simulink library "cylindricalPack_58kwhr_30Q_fade"  (R2025a)
settings: Solver=VariableStepAuto  StartTime=0.0  StopTime=10.0  RelTol=1e-3
undefined symbols (not defined in the file or in its folder): battery_builder_rtmsupport, gcbh
libraries: nesl_utility x75, cylindricalPack_58kwhr_30Q_fade_lib x36, batt_lib x1
(part 1 of 5)
settings Model: Creator=OADEBAJO  LastModifiedBy=OADEBAJO

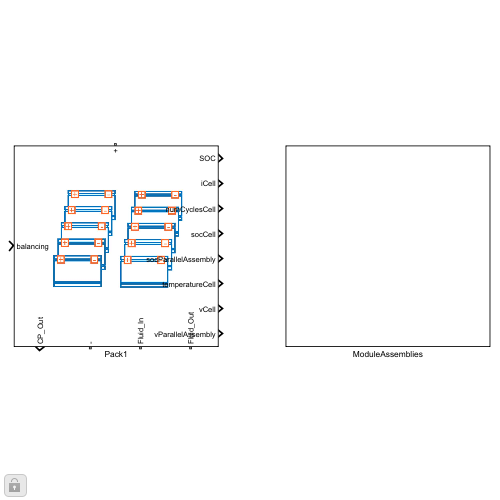
[thumbnail: Simulink's stored preview of the top-level diagram]
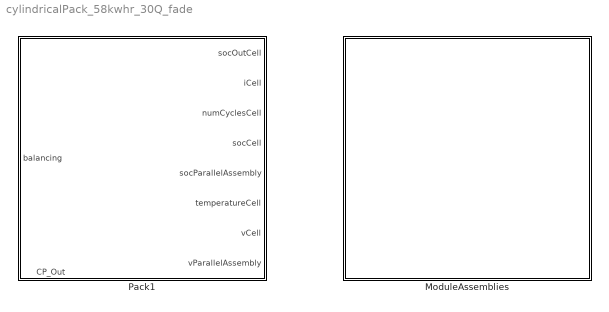
== system cylindricalPack_58kwhr_30Q_fade ==
  ModuleAssemblies : Subsystem
  Pack1 : Subsystem  LoadFcn=battery_builder_rtmsupport('loadfcn',gcbh);
      settings: CopyFcn=battery_builder_rtmsupport('copyfcn',gcbh);  PreCopyFcn=battery_builder_rtmsupport('precopyfcn',gcbh);  PreDeleteFcn=battery_builder_rtmsupport('predeletefcn',gcbh);  PortSchema="{\"entries\":[{\"content\":{\"sides\":[{\"content\":{\"connectorIds\":[\"LConn1\"]},\"type\":\"ConnectorPlacement.EquallySpacedRectSide\",\"uuid\":\"39220b85-9e56-421f-be99-25ff5c21c9d0\"},{\"content\":{\"connectorIds\":[\"Out1\",\"RConn1\",\"RConn2\",\"RConn3\"],\"side\":\"RIGHT\"},\"type\":\"ConnectorPlacement.EquallySpacedRectSide\",\"uuid\":\"8e68bd29-cf5f-450c-8507-e6fdf573813e\"},{\"content\":{\"connectorIds\":[\"In1\"],\"side\":\"TOP\"},\"type\":\"ConnectorPlacement.EquallySpacedRectSide\",\"uuid\":\"da231d6b-72d6-4d7b-b077-15d78428412a\"},{\"content\":{\"connectorIds\":[\"Out2\",\"Out3\",\"Out4\",\"Out5\",\"Out6\",\"Out7\",\"Out8\",\"Out9\"],\"side\":\"BOTTOM\"},\"type\":\"ConnectorPlacement.EquallySpacedRectSide\",\"uuid\":\"e98dc27c-cbdf-44be-82a1-87ffd4deded9\"}]},\"type\":\"ConnectorPlacement.EquallySpacedConnector\",\"uuid\":\"6b91b769-9080-486f-8a83-717e958640da\"}],\"packageUris\":[\"http://schema.mathworks.com/mf0/Connector/R2020b\"],\"version\":\"1.0\"}"
      mask Display: image('$imagefile')

== system cylindricalPack_58kwhr_30Q_fade/ModuleAssemblies ==
  ModuleAssemblyType1 : Subsystem  LoadFcn=battery_builder_rtmsupport('loadfcn',gcbh);
      settings: CopyFcn=battery_builder_rtmsupport('copyfcn',gcbh);  PreCopyFcn=battery_builder_rtmsupport('precopyfcn',gcbh);  PreDeleteFcn=battery_builder_rtmsupport('predeletefcn',gcbh);  PortSchema="{\"entries\":[{\"content\":{\"sides\":[{\"content\":{\"connectorIds\":[\"LConn1\"]},\"type\":\"ConnectorPlacement.EquallySpacedRectSide\",\"uuid\":\"edb2725c-ca29-40a6-9f70-0dabec9a46f5\"},{\"content\":{\"connectorIds\":[\"RConn1\",\"RConn2\"],\"side\":\"RIGHT\"},\"type\":\"ConnectorPlacement.EquallySpacedRectSide\",\"uuid\":\"4c0fe347-b718-4785-8871-63deed9ddb14\"},{\"content\":{\"connectorIds\":[\"In1\"],\"side\":\"TOP\"},\"type\":\"ConnectorPlacement.EquallySpacedRectSide\",\"uuid\":\"14c89690-db7b-421c-9ae6-2a7930fd5502\"},{\"content\":{\"connectorIds\":[\"Out1\",\"Out2\",\"Out3\",\"Out4\",\"Out5\",\"Out6\",\"Out7\",\"Out8\"],\"side\":\"BOTTOM\"},\"type\":\"ConnectorPlacement.EquallySpacedRectSide\",\"uuid\":\"cd90e9e9-4011-4b4d-baa7-3772b10580cf\"}]},\"type\":\"ConnectorPlacement.EquallySpacedConnector\",\"uuid\":\"bac0a601-b4a1-4bc6-ad24-9e7613281f89\"}],\"packageUris\":[\"http://schema.mathworks.com/mf0/Connector/R2020b\"],\"version\":\"1.0\"}"
      mask Display: image('$imagefile')
  ModuleAssemblyType2 : Subsystem  LoadFcn=battery_builder_rtmsupport('loadfcn',gcbh);
      settings: CopyFcn=battery_builder_rtmsupport('copyfcn',gcbh);  PreCopyFcn=battery_builder_rtmsupport('precopyfcn',gcbh);  PreDeleteFcn=battery_builder_rtmsupport('predeletefcn',gcbh);  PortSchema="{\"entries\":[{\"content\":{\"sides\":[{\"content\":{\"connectorIds\":[\"LConn1\"]},\"type\":\"ConnectorPlacement.EquallySpacedRectSide\",\"uuid\":\"edb2725c-ca29-40a6-9f70-0dabec9a46f5\"},{\"content\":{\"connectorIds\":[\"RConn1\",\"RConn2\"],\"side\":\"RIGHT\"},\"type\":\"ConnectorPlacement.EquallySpacedRectSide\",\"uuid\":\"4c0fe347-b718-4785-8871-63deed9ddb14\"},{\"content\":{\"connectorIds\":[\"In1\"],\"side\":\"TOP\"},\"type\":\"ConnectorPlacement.EquallySpacedRectSide\",\"uuid\":\"14c89690-db7b-421c-9ae6-2a7930fd5502\"},{\"content\":{\"connectorIds\":[\"Out1\",\"Out2\",\"Out3\",\"Out4\",\"Out5\",\"Out6\",\"Out7\",\"Out8\"],\"side\":\"BOTTOM\"},\"type\":\"ConnectorPlacement.EquallySpacedRectSide\",\"uuid\":\"26263ffa-138f-48ba-a92f-43b1044b6511\"}]},\"type\":\"ConnectorPlacement.EquallySpacedConnector\",\"uuid\":\"bac0a601-b4a1-4bc6-ad24-9e7613281f89\"}],\"packageUris\":[\"http://schema.mathworks.com/mf0/Connector/R2020b\"],\"version\":\"1.0\"}"
      mask Display: image('$imagefile')

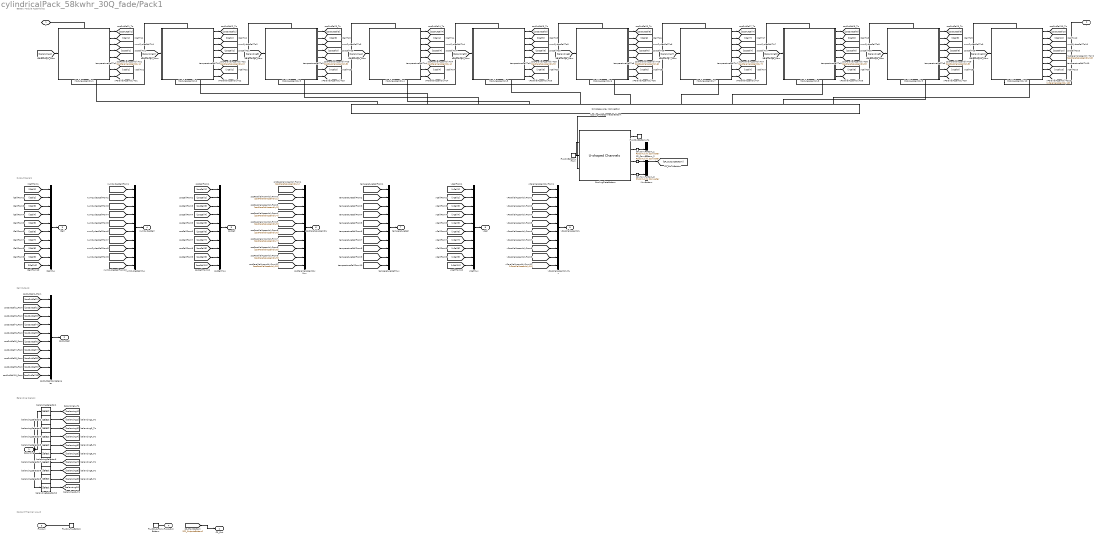
== system cylindricalPack_58kwhr_30Q_fade/Pack1 ==
  note: Battery Module Assemblies
  note: Output Signals
  note: Cell Outputs
  note: Balancing Signals
  note: Coolant Thermal Liquid
  balancing : Inport  PortDimensions=180
  CP_ConvBottom_1 : nesl_utility/PS-Simulink Converter  PhysicalDomain=network_engine_domain  SubClassName=ps_output  LeftPortType=input  RightPortType=output  PseudoPeriodic=off  Frequencies=[]  VectorFormat=inherit  Unit=inherit  AffineConversion=off
  CP_ConvBottom_2 : nesl_utility/PS-Simulink Converter  PhysicalDomain=network_engine_domain  SubClassName=ps_output  LeftPortType=input  RightPortType=output  PseudoPeriodic=off  Frequencies=[]  VectorFormat=inherit  Unit=inherit  AffineConversion=off
  CP_ConvBottom_3 : nesl_utility/PS-Simulink Converter  PhysicalDomain=network_engine_domain  SubClassName=ps_output  LeftPortType=input  RightPortType=output  PseudoPeriodic=off  Frequencies=[]  VectorFormat=inherit  Unit=inherit  AffineConversion=off
  CoolingPlateBottom : batt_lib/Thermal/U-shaped Channels  plateConnectivity=simscape.battery.enum.thermal.coolingPlateConnectivity.singleSided  numBattThermalNodes1=30  dimensionThermalNodes1=[[0.0955 0.7388;0.0955 0.7388;0.0955 0.7388;0.0955 0.7388;0.0955 0.7388;0.0955 0.7388;0.0955 0.7388;0.0955 0.7388;0.0955 0.7388;0.0955 0.7388;0.0955 0.7388;0.0955 0.7388;0.0955 0.7388;0.0955 0.7388;0.0955 0.7388;0.0955 0.7388;0.0955 0.7388;0.0955 0.7388;0.0955 0.7388;0.0955 0.7388;0.0955 0.7388;0.0955 0.7388;0.0955 0.7388;0.0955 0.7388;0.0955 0.7388;0.0955 0.7388;0.0955 0.7388;0.0955 0.7388;0.0955 0.7388;0.0955 0.7388]]  locationThermalNodes1=[[0.04775 0.3694;0.04775 0.3694;0.04775 0.3694;0.15325 0.3694;0.15325 0.3694;0.15325 0.3694;0.25875 0.3694;0.25875 0.3694;0.25875 0.3694;0.36425 0.3694;0.36425 0.3694;0.36425 0.3694;0.46975 0.3694;0.46975 0.3694;0.46975 0.3694;0.57525 0.3694;0.57525 0.3694;0.57525 0.3694;0.68075 0.3694;0.68075 0.3694;0.68075 0.3694;0.78625 0.3694;0.78625 0.3694;0.78625 0.3694;0.89175 0.3694;0.89175 0.3694;0.89175 0.3694;0.99725 0.3694;0.99725 0.3694;0.99725 0.3694]]  numBattThermalNodes2=1  dimensionThermalNodes2=ones(1, 2)  locationThermalNodes2=ones(1, 2)  plateDimX=2  plateDimY=5  plateTh=2e-3 m  plateThCond=20 W/(K*m)  plateDen=2500 kg/m^3  plateCp=447 J/(K*kg)  plateTemp_ini=300 K  Re_lam=2000  Re_tur=4000  Nu_lam=3.66  length_add=1e-3 m  shape_factor=64  nPartitions=1  selectChannelOrientation=simscape.battery.enum.thermal.coolingChannelsDirection.alongX  channelThickness=5e-03 m  barrierWidth=5e-03 m  roughnessPipe=1.5e-05 m
      settings: InternalSimscapePortConfiguration="{\"Bottom\":[],\"Left\":[{\"id\":\"fluid_in\",\"label\":\"fluid_in\",\"type\":\"foundation.thermal_liquid.thermal_liquid\"}],\"Right\":[{\"id\":\"fluid_out\",\"label\":\"fluid_out\",\"type\":\"foundation.thermal_liquid.thermal_liquid\"},{\"id\":\"plotPlateT\",\"label\":\"Tp\",\"type\":\"output\"},{\"id\":\"tempSensor\",\"label\":\"dT\",\"type\":\"output\"},{\"id\":\"presSensor\",\"label\":\"dP\",\"type\":\"output\"}],\"Top\":[{\"id\":\"Side1\",\"label\":\"Surf1\",\"type\":\"foundation.thermal.thermal\"}]}"
  CoolingPlateConnectorBottom : SimscapeArrayConnection  Domain=foundation.thermal.thermal  Mode=Sized Elements
  FluidInBottom_From : ConnectionLabel  Label=FluidIn_To_Bottom
  FluidIn_To_Bottom : ConnectionLabel  Label=FluidIn_To_Bottom
  FluidOutBottom_To : ConnectionLabel  Label=FluidOut_From_Bottom
  FluidOut_From_Bottom : ConnectionLabel  Label=FluidOut_From_Bottom
  ModuleAssembly1 : Subsystem  LoadFcn=battery_builder_rtmsupport('loadfcn',gcbh);
      settings: CopyFcn=battery_builder_rtmsupport('copyfcn',gcbh);  PreCopyFcn=battery_builder_rtmsupport('precopyfcn',gcbh);  PreDeleteFcn=battery_builder_rtmsupport('predeletefcn',gcbh);  PortSchema="{\"entries\":[{\"content\":{\"sides\":[{\"content\":{\"connectorIds\":[\"LConn1\"]},\"type\":\"ConnectorPlacement.EquallySpacedRectSide\",\"uuid\":\"edb2725c-ca29-40a6-9f70-0dabec9a46f5\"},{\"content\":{\"connectorIds\":[\"RConn1\",\"RConn2\"],\"side\":\"RIGHT\"},\"type\":\"ConnectorPlacement.EquallySpacedRectSide\",\"uuid\":\"4c0fe347-b718-4785-8871-63deed9ddb14\"},{\"content\":{\"connectorIds\":[\"In1\"],\"side\":\"TOP\"},\"type\":\"ConnectorPlacement.EquallySpacedRectSide\",\"uuid\":\"14c89690-db7b-421c-9ae6-2a7930fd5502\"},{\"content\":{\"connectorIds\":[\"Out1\",\"Out2\",\"Out3\",\"Out4\",\"Out5\",\"Out6\",\"Out7\",\"Out8\"],\"side\":\"BOTTOM\"},\"type\":\"ConnectorPlacement.EquallySpacedRectSide\",\"uuid\":\"cd90e9e9-4011-4b4d-baa7-3772b10580cf\"}]},\"type\":\"ConnectorPlacement.EquallySpacedConnector\",\"uuid\":\"bac0a601-b4a1-4bc6-ad24-9e7613281f89\"}],\"packageUris\":[\"http://schema.mathworks.com/mf0/Connector/R2020b\"],\"version\":\"1.0\"}"
      mask Display: image('$imagefile')
  ModuleAssembly10 : Subsystem  LoadFcn=battery_builder_rtmsupport('loadfcn',gcbh);
      settings: CopyFcn=battery_builder_rtmsupport('copyfcn',gcbh);  PreCopyFcn=battery_builder_rtmsupport('precopyfcn',gcbh);  PreDeleteFcn=battery_builder_rtmsupport('predeletefcn',gcbh);  PortSchema="{\"entries\":[{\"content\":{\"sides\":[{\"content\":{\"connectorIds\":[\"LConn1\"]},\"type\":\"ConnectorPlacement.EquallySpacedRectSide\",\"uuid\":\"edb2725c-ca29-40a6-9f70-0dabec9a46f5\"},{\"content\":{\"connectorIds\":[\"RConn1\",\"RConn2\"],\"side\":\"RIGHT\"},\"type\":\"ConnectorPlacement.EquallySpacedRectSide\",\"uuid\":\"4c0fe347-b718-4785-8871-63deed9ddb14\"},{\"content\":{\"connectorIds\":[\"In1\"],\"side\":\"TOP\"},\"type\":\"ConnectorPlacement.EquallySpacedRectSide\",\"uuid\":\"14c89690-db7b-421c-9ae6-2a7930fd5502\"},{\"content\":{\"connectorIds\":[\"Out1\",\"Out2\",\"Out3\",\"Out4\",\"Out5\",\"Out6\",\"Out7\",\"Out8\"],\"side\":\"BOTTOM\"},\"type\":\"ConnectorPlacement.EquallySpacedRectSide\",\"uuid\":\"26263ffa-138f-48ba-a92f-43b1044b6511\"}]},\"type\":\"ConnectorPlacement.EquallySpacedConnector\",\"uuid\":\"bac0a601-b4a1-4bc6-ad24-9e7613281f89\"}],\"packageUris\":[\"http://schema.mathworks.com/mf0/Connector/R2020b\"],\"version\":\"1.0\"}"
      mask Display: image('$imagefile')
  ModuleAssembly2 : Subsystem  LoadFcn=battery_builder_rtmsupport('loadfcn',gcbh);
      settings: CopyFcn=battery_builder_rtmsupport('copyfcn',gcbh);  PreCopyFcn=battery_builder_rtmsupport('precopyfcn',gcbh);  PreDeleteFcn=battery_builder_rtmsupport('predeletefcn',gcbh);  PortSchema="{\"entries\":[{\"content\":{\"sides\":[{\"content\":{\"connectorIds\":[\"LConn1\"]},\"type\":\"ConnectorPlacement.EquallySpacedRectSide\",\"uuid\":\"edb2725c-ca29-40a6-9f70-0dabec9a46f5\"},{\"content\":{\"connectorIds\":[\"RConn1\",\"RConn2\"],\"side\":\"RIGHT\"},\"type\":\"ConnectorPlacement.EquallySpacedRectSide\",\"uuid\":\"4c0fe347-b718-4785-8871-63deed9ddb14\"},{\"content\":{\"connectorIds\":[\"In1\"],\"side\":\"TOP\"},\"type\":\"ConnectorPlacement.EquallySpacedRectSide\",\"uuid\":\"14c89690-db7b-421c-9ae6-2a7930fd5502\"},{\"content\":{\"connectorIds\":[\"Out1\",\"Out2\",\"Out3\",\"Out4\",\"Out5\",\"Out6\",\"Out7\",\"Out8\"],\"side\":\"BOTTOM\"},\"type\":\"ConnectorPlacement.EquallySpacedRectSide\",\"uuid\":\"26263ffa-138f-48ba-a92f-43b1044b6511\"}]},\"type\":\"ConnectorPlacement.EquallySpacedConnector\",\"uuid\":\"bac0a601-b4a1-4bc6-ad24-9e7613281f89\"}],\"packageUris\":[\"http://schema.mathworks.com/mf0/Connector/R2020b\"],\"version\":\"1.0\"}"
      mask Display: image('$imagefile')
  ModuleAssembly3 : Subsystem  LoadFcn=battery_builder_rtmsupport('loadfcn',gcbh);
      settings: CopyFcn=battery_builder_rtmsupport('copyfcn',gcbh);  PreCopyFcn=battery_builder_rtmsupport('precopyfcn',gcbh);  PreDeleteFcn=battery_builder_rtmsupport('predeletefcn',gcbh);  PortSchema="{\"entries\":[{\"content\":{\"sides\":[{\"content\":{\"connectorIds\":[\"LConn1\"]},\"type\":\"ConnectorPlacement.EquallySpacedRectSide\",\"uuid\":\"edb2725c-ca29-40a6-9f70-0dabec9a46f5\"},{\"content\":{\"connectorIds\":[\"RConn1\",\"RConn2\"],\"side\":\"RIGHT\"},\"type\":\"ConnectorPlacement.EquallySpacedRectSide\",\"uuid\":\"4c0fe347-b718-4785-8871-63deed9ddb14\"},{\"content\":{\"connectorIds\":[\"In1\"],\"side\":\"TOP\"},\"type\":\"ConnectorPlacement.EquallySpacedRectSide\",\"uuid\":\"14c89690-db7b-421c-9ae6-2a7930fd5502\"},{\"content\":{\"connectorIds\":[\"Out1\",\"Out2\",\"Out3\",\"Out4\",\"Out5\",\"Out6\",\"Out7\",\"Out8\"],\"side\":\"BOTTOM\"},\"type\":\"ConnectorPlacement.EquallySpacedRectSide\",\"uuid\":\"26263ffa-138f-48ba-a92f-43b1044b6511\"}]},\"type\":\"ConnectorPlacement.EquallySpacedConnector\",\"uuid\":\"bac0a601-b4a1-4bc6-ad24-9e7613281f89\"}],\"packageUris\":[\"http://schema.mathworks.com/mf0/Connector/R2020b\"],\"version\":\"1.0\"}"
      mask Display: image('$imagefile')
  ModuleAssembly4 : Subsystem  LoadFcn=battery_builder_rtmsupport('loadfcn',gcbh);
      settings: CopyFcn=battery_builder_rtmsupport('copyfcn',gcbh);  PreCopyFcn=battery_builder_rtmsupport('precopyfcn',gcbh);  PreDeleteFcn=battery_builder_rtmsupport('predeletefcn',gcbh);  PortSchema="{\"entries\":[{\"content\":{\"sides\":[{\"content\":{\"connectorIds\":[\"LConn1\"]},\"type\":\"ConnectorPlacement.EquallySpacedRectSide\",\"uuid\":\"edb2725c-ca29-40a6-9f70-0dabec9a46f5\"},{\"content\":{\"connectorIds\":[\"RConn1\",\"RConn2\"],\"side\":\"RIGHT\"},\"type\":\"ConnectorPlacement.EquallySpacedRectSide\",\"uuid\":\"4c0fe347-b718-4785-8871-63deed9ddb14\"},{\"content\":{\"connectorIds\":[\"In1\"],\"side\":\"TOP\"},\"type\":\"ConnectorPlacement.EquallySpacedRectSide\",\"uuid\":\"14c89690-db7b-421c-9ae6-2a7930fd5502\"},{\"content\":{\"connectorIds\":[\"Out1\",\"Out2\",\"Out3\",\"Out4\",\"Out5\",\"Out6\",\"Out7\",\"Out8\"],\"side\":\"BOTTOM\"},\"type\":\"ConnectorPlacement.EquallySpacedRectSide\",\"uuid\":\"26263ffa-138f-48ba-a92f-43b1044b6511\"}]},\"type\":\"ConnectorPlacement.EquallySpacedConnector\",\"uuid\":\"bac0a601-b4a1-4bc6-ad24-9e7613281f89\"}],\"packageUris\":[\"http://schema.mathworks.com/mf0/Connector/R2020b\"],\"version\":\"1.0\"}"
      mask Display: image('$imagefile')
  ModuleAssembly5 : Subsystem  LoadFcn=battery_builder_rtmsupport('loadfcn',gcbh);
      settings: CopyFcn=battery_builder_rtmsupport('copyfcn',gcbh);  PreCopyFcn=battery_builder_rtmsupport('precopyfcn',gcbh);  PreDeleteFcn=battery_builder_rtmsupport('predeletefcn',gcbh);  PortSchema="{\"entries\":[{\"content\":{\"sides\":[{\"content\":{\"connectorIds\":[\"LConn1\"]},\"type\":\"ConnectorPlacement.EquallySpacedRectSide\",\"uuid\":\"edb2725c-ca29-40a6-9f70-0dabec9a46f5\"},{\"content\":{\"connectorIds\":[\"RConn1\",\"RConn2\"],\"side\":\"RIGHT\"},\"type\":\"ConnectorPlacement.EquallySpacedRectSide\",\"uuid\":\"4c0fe347-b718-4785-8871-63deed9ddb14\"},{\"content\":{\"connectorIds\":[\"In1\"],\"side\":\"TOP\"},\"type\":\"ConnectorPlacement.EquallySpacedRectSide\",\"uuid\":\"14c89690-db7b-421c-9ae6-2a7930fd5502\"},{\"content\":{\"connectorIds\":[\"Out1\",\"Out2\",\"Out3\",\"Out4\",\"Out5\",\"Out6\",\"Out7\",\"Out8\"],\"side\":\"BOTTOM\"},\"type\":\"ConnectorPlacement.EquallySpacedRectSide\",\"uuid\":\"26263ffa-138f-48ba-a92f-43b1044b6511\"}]},\"type\":\"ConnectorPlacement.EquallySpacedConnector\",\"uuid\":\"bac0a601-b4a1-4bc6-ad24-9e7613281f89\"}],\"packageUris\":[\"http://schema.mathworks.com/mf0/Connector/R2020b\"],\"version\":\"1.0\"}"
      mask Display: image('$imagefile')
  ModuleAssembly6 : Subsystem  LoadFcn=battery_builder_rtmsupport('loadfcn',gcbh);
      settings: CopyFcn=battery_builder_rtmsupport('copyfcn',gcbh);  PreCopyFcn=battery_builder_rtmsupport('precopyfcn',gcbh);  PreDeleteFcn=battery_builder_rtmsupport('predeletefcn',gcbh);  PortSchema="{\"entries\":[{\"content\":{\"sides\":[{\"content\":{\"connectorIds\":[\"LConn1\"]},\"type\":\"ConnectorPlacement.EquallySpacedRectSide\",\"uuid\":\"edb2725c-ca29-40a6-9f70-0dabec9a46f5\"},{\"content\":{\"connectorIds\":[\"RConn1\",\"RConn2\"],\"side\":\"RIGHT\"},\"type\":\"ConnectorPlacement.EquallySpacedRectSide\",\"uuid\":\"4c0fe347-b718-4785-8871-63deed9ddb14\"},{\"content\":{\"connectorIds\":[\"In1\"],\"side\":\"TOP\"},\"type\":\"ConnectorPlacement.EquallySpacedRectSide\",\"uuid\":\"14c89690-db7b-421c-9ae6-2a7930fd5502\"},{\"content\":{\"connectorIds\":[\"Out1\",\"Out2\",\"Out3\",\"Out4\",\"Out5\",\"Out6\",\"Out7\",\"Out8\"],\"side\":\"BOTTOM\"},\"type\":\"ConnectorPlacement.EquallySpacedRectSide\",\"uuid\":\"26263ffa-138f-48ba-a92f-43b1044b6511\"}]},\"type\":\"ConnectorPlacement.EquallySpacedConnector\",\"uuid\":\"bac0a601-b4a1-4bc6-ad24-9e7613281f89\"}],\"packageUris\":[\"http://schema.mathworks.com/mf0/Connector/R2020b\"],\"version\":\"1.0\"}"
      mask Display: image('$imagefile')
  ModuleAssembly7 : Subsystem  LoadFcn=battery_builder_rtmsupport('loadfcn',gcbh);
      settings: CopyFcn=battery_builder_rtmsupport('copyfcn',gcbh);  PreCopyFcn=battery_builder_rtmsupport('precopyfcn',gcbh);  PreDeleteFcn=battery_builder_rtmsupport('predeletefcn',gcbh);  PortSchema="{\"entries\":[{\"content\":{\"sides\":[{\"content\":{\"connectorIds\":[\"LConn1\"]},\"type\":\"ConnectorPlacement.EquallySpacedRectSide\",\"uuid\":\"edb2725c-ca29-40a6-9f70-0dabec9a46f5\"},{\"content\":{\"connectorIds\":[\"RConn1\",\"RConn2\"],\"side\":\"RIGHT\"},\"type\":\"ConnectorPlacement.EquallySpacedRectSide\",\"uuid\":\"4c0fe347-b718-4785-8871-63deed9ddb14\"},{\"content\":{\"connectorIds\":[\"In1\"],\"side\":\"TOP\"},\"type\":\"ConnectorPlacement.EquallySpacedRectSide\",\"uuid\":\"14c89690-db7b-421c-9ae6-2a7930fd5502\"},{\"content\":{\"connectorIds\":[\"Out1\",\"Out2\",\"Out3\",\"Out4\",\"Out5\",\"Out6\",\"Out7\",\"Out8\"],\"side\":\"BOTTOM\"},\"type\":\"ConnectorPlacement.EquallySpacedRectSide\",\"uuid\":\"26263ffa-138f-48ba-a92f-43b1044b6511\"}]},\"type\":\"ConnectorPlacement.EquallySpacedConnector\",\"uuid\":\"bac0a601-b4a1-4bc6-ad24-9e7613281f89\"}],\"packageUris\":[\"http://schema.mathworks.com/mf0/Connector/R2020b\"],\"version\":\"1.0\"}"
      mask Display: image('$imagefile')
  ModuleAssembly8 : Subsystem  LoadFcn=battery_builder_rtmsupport('loadfcn',gcbh);
      settings: CopyFcn=battery_builder_rtmsupport('copyfcn',gcbh);  PreCopyFcn=battery_builder_rtmsupport('precopyfcn',gcbh);  PreDeleteFcn=battery_builder_rtmsupport('predeletefcn',gcbh);  PortSchema="{\"entries\":[{\"content\":{\"sides\":[{\"content\":{\"connectorIds\":[\"LConn1\"]},\"type\":\"ConnectorPlacement.EquallySpacedRectSide\",\"uuid\":\"edb2725c-ca29-40a6-9f70-0dabec9a46f5\"},{\"content\":{\"connectorIds\":[\"RConn1\",\"RConn2\"],\"side\":\"RIGHT\"},\"type\":\"ConnectorPlacement.EquallySpacedRectSide\",\"uuid\":\"4c0fe347-b718-4785-8871-63deed9ddb14\"},{\"content\":{\"connectorIds\":[\"In1\"],\"side\":\"TOP\"},\"type\":\"ConnectorPlacement.EquallySpacedRectSide\",\"uuid\":\"14c89690-db7b-421c-9ae6-2a7930fd5502\"},{\"content\":{\"connectorIds\":[\"Out1\",\"Out2\",\"Out3\",\"Out4\",\"Out5\",\"Out6\",\"Out7\",\"Out8\"],\"side\":\"BOTTOM\"},\"type\":\"ConnectorPlacement.EquallySpacedRectSide\",\"uuid\":\"26263ffa-138f-48ba-a92f-43b1044b6511\"}]},\"type\":\"ConnectorPlacement.EquallySpacedConnector\",\"uuid\":\"bac0a601-b4a1-4bc6-ad24-9e7613281f89\"}],\"packageUris\":[\"http://schema.mathworks.com/mf0/Connector/R2020b\"],\"version\":\"1.0\"}"
      mask Display: image('$imagefile')
  ModuleAssembly9 : Subsystem  LoadFcn=battery_builder_rtmsupport('loadfcn',gcbh);
      settings: CopyFcn=battery_builder_rtmsupport('copyfcn',gcbh);  PreCopyFcn=battery_builder_rtmsupport('precopyfcn',gcbh);  PreDeleteFcn=battery_builder_rtmsupport('predeletefcn',gcbh);  PortSchema="{\"entries\":[{\"content\":{\"sides\":[{\"content\":{\"connectorIds\":[\"LConn1\"]},\"type\":\"ConnectorPlacement.EquallySpacedRectSide\",\"uuid\":\"edb2725c-ca29-40a6-9f70-0dabec9a46f5\"},{\"content\":{\"connectorIds\":[\"RConn1\",\"RConn2\"],\"side\":\"RIGHT\"},\"type\":\"ConnectorPlacement.EquallySpacedRectSide\",\"uuid\":\"4c0fe347-b718-4785-8871-63deed9ddb14\"},{\"content\":{\"connectorIds\":[\"In1\"],\"side\":\"TOP\"},\"type\":\"ConnectorPlacement.EquallySpacedRectSide\",\"uuid\":\"14c89690-db7b-421c-9ae6-2a7930fd5502\"},{\"content\":{\"connectorIds\":[\"Out1\",\"Out2\",\"Out3\",\"Out4\",\"Out5\",\"Out6\",\"Out7\",\"Out8\"],\"side\":\"BOTTOM\"},\"type\":\"ConnectorPlacement.EquallySpacedRectSide\",\"uuid\":\"26263ffa-138f-48ba-a92f-43b1044b6511\"}]},\"type\":\"ConnectorPlacement.EquallySpacedConnector\",\"uuid\":\"bac0a601-b4a1-4bc6-ad24-9e7613281f89\"}],\"packageUris\":[\"http://schema.mathworks.com/mf0/Connector/R2020b\"],\"version\":\"1.0\"}"
      mask Display: image('$imagefile')
  MuxBottom : Mux  Inputs=3
  balancingSelector1 : Selector  InputPortWidth=180  IndexOptions=Index vector (dialog)  Indices="[1   2   3   4   5   6   7   8   9  10  11  12  13  14  15  16  17  18]"  OutputSizes=1
  balancingSelector10 : Selector  InputPortWidth=180  IndexOptions=Index vector (dialog)  Indices="[163  164  165  166  167  168  169  170  171  172  173  174  175  176  177  178  179  180]"  OutputSizes=1
  balancingSelector2 : Selector  InputPortWidth=180  IndexOptions=Index vector (dialog)  Indices="[19  20  21  22  23  24  25  26  27  28  29  30  31  32  33  34  35  36]"  OutputSizes=1
  balancingSelector3 : Selector  InputPortWidth=180  IndexOptions=Index vector (dialog)  Indices="[37  38  39  40  41  42  43  44  45  46  47  48  49  50  51  52  53  54]"  OutputSizes=1
  balancingSelector4 : Selector  InputPortWidth=180  IndexOptions=Index vector (dialog)  Indices="[55  56  57  58  59  60  61  62  63  64  65  66  67  68  69  70  71  72]"  OutputSizes=1
  balancingSelector5 : Selector  InputPortWidth=180  IndexOptions=Index vector (dialog)  Indices="[73  74  75  76  77  78  79  80  81  82  83  84  85  86  87  88  89  90]"  OutputSizes=1
  balancingSelector6 : Selector  InputPortWidth=180  IndexOptions=Index vector (dialog)  Indices="[91   92   93   94   95   96   97   98   99  100  101  102  103  104  105  106  107  108]"  OutputSizes=1
  balancingSelector7 : Selector  InputPortWidth=180  IndexOptions=Index vector (dialog)  Indices="[109  110  111  112  113  114  115  116  117  118  119  120  121  122  123  124  125  126]"  OutputSizes=1
  balancingSelector8 : Selector  InputPortWidth=180  IndexOptions=Index vector (dialog)  Indices="[127  128  129  130  131  132  133  134  135  136  137  138  139  140  141  142  143  144]"  OutputSizes=1
  balancingSelector9 : Selector  InputPortWidth=180  IndexOptions=Index vector (dialog)  Indices="[145  146  147  148  149  150  151  152  153  154  155  156  157  158  159  160  161  162]"  OutputSizes=1
  iCellMux : Mux  Inputs=10
  numCyclesCellMux : Mux  Inputs=10
  socCellMux : Mux  Inputs=10
  socOutCellConcatenate : Concatenate  NumInputs=10  Mode=Multidimensional array  ConcatenateDimension=2
  socParallelAssemblyMux : Mux  Inputs=10
  temperatureCellMux : Mux  Inputs=10
  vCellMux : Mux  Inputs=10
  vParallelAssemblyMux : Mux  Inputs=10
  + : PMIOPort  Side=Left
  - : PMIOPort  Port=2  Side=Right
  Fluid_In : PMIOPort  Port=3  Side=Right  ConnectionType=Connection: foundation.thermal_liquid.thermal_liquid
  Fluid_Out : PMIOPort  Port=4  Side=Right  ConnectionType=Connection: foundation.thermal_liquid.thermal_liquid
  CP_Out : Outport
  socOutCell : Outport  Port=2
  iCell : Outport  Port=3
  numCyclesCell : Outport  Port=4
  socCell : Outport  Port=5
  socParallelAssembly : Outport  Port=6
  temperatureCell : Outport  Port=7
  vCell : Outport  Port=8
  vParallelAssembly : Outport  Port=9
  wires:
  socOutCellConcatenate/1 -> socOutCell/1  "SOC"
  [socOutCell1] -> socOutCellConcatenate/1
  [socOutCell2] -> socOutCellConcatenate/2
  [socOutCell3] -> socOutCellConcatenate/3
  [socOutCell4] -> socOutCellConcatenate/4
  [socOutCell5] -> socOutCellConcatenate/5
  [socOutCell6] -> socOutCellConcatenate/6
  [socOutCell7] -> socOutCellConcatenate/7
  [socOutCell8] -> socOutCellConcatenate/8
  [socOutCell9] -> socOutCellConcatenate/9
  [socOutCell10] -> socOutCellConcatenate/10
  ModuleAssembly1/2(iCell) -> [iCell1]
  iCellMux/1 -> iCell/1
  [iCell1] -> iCellMux/1
  ModuleAssembly1/3(numCyclesCell) -> [numCyclesCell1]
  numCyclesCellMux/1 -> numCyclesCell/1
  [numCyclesCell1] -> numCyclesCellMux/1
  ModuleAssembly1/4(socCell) -> [socCell1]
  socCellMux/1 -> socCell/1
  [socCell1] -> socCellMux/1
  ModuleAssembly1/5(socParallelAssembly) -> [socParallelAssembly1]
  socParallelAssemblyMux/1 -> socParallelAssembly/1
  [socParallelAssembly1] -> socParallelAssemblyMux/1
  ModuleAssembly1/6(temperatureCell) -> [temperatureCell1]
  temperatureCellMux/1 -> temperatureCell/1
  [temperatureCell1] -> temperatureCellMux/1
  ModuleAssembly1/7(vCell) -> [vCell1]
  vCellMux/1 -> vCell/1
  [vCell1] -> vCellMux/1
  ModuleAssembly1/8(vParallelAssembly) -> [vParallelAssembly1]
  vParallelAssemblyMux/1 -> vParallelAssembly/1
  [vParallelAssembly1] -> vParallelAssemblyMux/1
  ModuleAssembly2/2(iCell) -> [iCell2]
  [iCell2] -> iCellMux/2
  ModuleAssembly2/3(numCyclesCell) -> [numCyclesCell2]
  [numCyclesCell2] -> numCyclesCellMux/2
  ModuleAssembly2/4(socCell) -> [socCell2]
  [socCell2] -> socCellMux/2
  ModuleAssembly2/5(socParallelAssembly) -> [socParallelAssembly2]
  [socParallelAssembly2] -> socParallelAssemblyMux/2
  ModuleAssembly2/6(temperatureCell) -> [temperatureCell2]
  [temperatureCell2] -> temperatureCellMux/2
  ModuleAssembly2/7(vCell) -> [vCell2]
  [vCell2] -> vCellMux/2
  ModuleAssembly2/8(vParallelAssembly) -> [vParallelAssembly2]
  [vParallelAssembly2] -> vParallelAssemblyMux/2
  ModuleAssembly3/2(iCell) -> [iCell3]
  [iCell3] -> iCellMux/3
  ModuleAssembly3/3(numCyclesCell) -> [numCyclesCell3]
  [numCyclesCell3] -> numCyclesCellMux/3
  ModuleAssembly3/4(socCell) -> [socCell3]
  [socCell3] -> socCellMux/3
  ModuleAssembly3/5(socParallelAssembly) -> [socParallelAssembly3]
  [socParallelAssembly3] -> socParallelAssemblyMux/3
  ModuleAssembly3/6(temperatureCell) -> [temperatureCell3]
  [temperatureCell3] -> temperatureCellMux/3
  ModuleAssembly3/7(vCell) -> [vCell3]
  [vCell3] -> vCellMux/3
  ModuleAssembly3/8(vParallelAssembly) -> [vParallelAssembly3]
  [vParallelAssembly3] -> vParallelAssemblyMux/3
  ModuleAssembly4/2(iCell) -> [iCell4]
  [iCell4] -> iCellMux/4
  ModuleAssembly4/3(numCyclesCell) -> [numCyclesCell4]
  [numCyclesCell4] -> numCyclesCellMux/4
  ModuleAssembly4/4(socCell) -> [socCell4]
  [socCell4] -> socCellMux/4
  ModuleAssembly4/5(socParallelAssembly) -> [socParallelAssembly4]
  [socParallelAssembly4] -> socParallelAssemblyMux/4
  ModuleAssembly4/6(temperatureCell) -> [temperatureCell4]
  [temperatureCell4] -> temperatureCellMux/4
  ModuleAssembly4/7(vCell) -> [vCell4]
  [vCell4] -> vCellMux/4
  ModuleAssembly4/8(vParallelAssembly) -> [vParallelAssembly4]
  [vParallelAssembly4] -> vParallelAssemblyMux/4
  ModuleAssembly5/2(iCell) -> [iCell5]
  [iCell5] -> iCellMux/5
  ModuleAssembly5/3(numCyclesCell) -> [numCyclesCell5]
  [numCyclesCell5] -> numCyclesCellMux/5
  ModuleAssembly5/4(socCell) -> [socCell5]
  [socCell5] -> socCellMux/5
  ModuleAssembly5/5(socParallelAssembly) -> [socParallelAssembly5]
  [socParallelAssembly5] -> socParallelAssemblyMux/5
  ModuleAssembly5/6(temperatureCell) -> [temperatureCell5]
  [temperatureCell5] -> temperatureCellMux/5
  ModuleAssembly5/7(vCell) -> [vCell5]
  [vCell5] -> vCellMux/5
  ModuleAssembly5/8(vParallelAssembly) -> [vParallelAssembly5]
  [vParallelAssembly5] -> vParallelAssemblyMux/5
  ModuleAssembly6/2(iCell) -> [iCell6]
  [iCell6] -> iCellMux/6
  ModuleAssembly6/3(numCyclesCell) -> [numCyclesCell6]
  [numCyclesCell6] -> numCyclesCellMux/6
  ModuleAssembly6/4(socCell) -> [socCell6]
  [socCell6] -> socCellMux/6
  ModuleAssembly6/5(socParallelAssembly) -> [socParallelAssembly6]
  [socParallelAssembly6] -> socParallelAssemblyMux/6
  ModuleAssembly6/6(temperatureCell) -> [temperatureCell6]
  [temperatureCell6] -> temperatureCellMux/6
  ModuleAssembly6/7(vCell) -> [vCell6]
  [vCell6] -> vCellMux/6
  ModuleAssembly6/8(vParallelAssembly) -> [vParallelAssembly6]
  [vParallelAssembly6] -> vParallelAssemblyMux/6
  ModuleAssembly7/2(iCell) -> [iCell7]
  [iCell7] -> iCellMux/7
  ModuleAssembly7/3(numCyclesCell) -> [numCyclesCell7]
  [numCyclesCell7] -> numCyclesCellMux/7
  ModuleAssembly7/4(socCell) -> [socCell7]
  [socCell7] -> socCellMux/7
  ModuleAssembly7/5(socParallelAssembly) -> [socParallelAssembly7]
  [socParallelAssembly7] -> socParallelAssemblyMux/7
  ModuleAssembly7/6(temperatureCell) -> [temperatureCell7]
  [temperatureCell7] -> temperatureCellMux/7
  ModuleAssembly7/7(vCell) -> [vCell7]
  [vCell7] -> vCellMux/7
  ModuleAssembly7/8(vParallelAssembly) -> [vParallelAssembly7]
  [vParallelAssembly7] -> vParallelAssemblyMux/7
  ModuleAssembly8/2(iCell) -> [iCell8]
  [iCell8] -> iCellMux/8
  ModuleAssembly8/3(numCyclesCell) -> [numCyclesCell8]
  [numCyclesCell8] -> numCyclesCellMux/8
  ModuleAssembly8/4(socCell) -> [socCell8]
  [socCell8] -> socCellMux/8
  ModuleAssembly8/5(socParallelAssembly) -> [socParallelAssembly8]
  [socParallelAssembly8] -> socParallelAssemblyMux/8
  ModuleAssembly8/6(temperatureCell) -> [temperatureCell8]
  [temperatureCell8] -> temperatureCellMux/8
  ModuleAssembly8/7(vCell) -> [vCell8]
  [vCell8] -> vCellMux/8
  ModuleAssembly8/8(vParallelAssembly) -> [vParallelAssembly8]
  [vParallelAssembly8] -> vParallelAssemblyMux/8
  ModuleAssembly9/2(iCell) -> [iCell9]
  [iCell9] -> iCellMux/9
  ModuleAssembly9/3(numCyclesCell) -> [numCyclesCell9]
  [numCyclesCell9] -> numCyclesCellMux/9
  ModuleAssembly9/4(socCell) -> [socCell9]
  [socCell9] -> socCellMux/9
  ModuleAssembly9/5(socParallelAssembly) -> [socParallelAssembly9]
  [socParallelAssembly9] -> socParallelAssemblyMux/9
  ModuleAssembly9/6(temperatureCell) -> [temperatureCell9]
  [temperatureCell9] -> temperatureCellMux/9
  ModuleAssembly9/7(vCell) -> [vCell9]
  [vCell9] -> vCellMux/9
  ModuleAssembly9/8(vParallelAssembly) -> [vParallelAssembly9]
  [vParallelAssembly9] -> vParallelAssemblyMux/9
  ModuleAssembly10/2(iCell) -> [iCell10]
  [iCell10] -> iCellMux/10
  ModuleAssembly10/3(numCyclesCell) -> [numCyclesCell10]
  [numCyclesCell10] -> numCyclesCellMux/10
  ModuleAssembly10/4(socCell) -> [socCell10]
  [socCell10] -> socCellMux/10
  ModuleAssembly10/5(socParallelAssembly) -> [socParallelAssembly10]
  [socParallelAssembly10] -> socParallelAssemblyMux/10
  ModuleAssembly10/6(temperatureCell) -> [temperatureCell10]
  [temperatureCell10] -> temperatureCellMux/10
  ModuleAssembly10/7(vCell) -> [vCell10]
  [vCell10] -> vCellMux/10
  ModuleAssembly10/8(vParallelAssembly) -> [vParallelAssembly10]
  [vParallelAssembly10] -> vParallelAssemblyMux/10
  ModuleAssembly1/1(socOutCell) -> [socOutCell1]
  ModuleAssembly2/1(socOutCell) -> [socOutCell2]
  ModuleAssembly3/1(socOutCell) -> [socOutCell3]
  ModuleAssembly4/1(socOutCell) -> [socOutCell4]
  ModuleAssembly5/1(socOutCell) -> [socOutCell5]
  ModuleAssembly6/1(socOutCell) -> [socOutCell6]
  ModuleAssembly7/1(socOutCell) -> [socOutCell7]
  ModuleAssembly8/1(socOutCell) -> [socOutCell8]
  ModuleAssembly9/1(socOutCell) -> [socOutCell9]
  ModuleAssembly10/1(socOutCell) -> [socOutCell10]
  [balancing1] -> ModuleAssembly1/1(balancing)
  balancing/1 -> balancingSelector1/1, balancingSelector2/1, balancingSelector3/1, balancingSelector4/1, balancingSelector5/1, balancingSelector6/1, balancingSelector7/1, balancingSelector8/1, balancingSelector9/1, balancingSelector10/1
  balancingSelector1/1 -> [balancing1]
  [balancing2] -> ModuleAssembly2/1(balancing)
  balancingSelector2/1 -> [balancing2]
  [balancing3] -> ModuleAssembly3/1(balancing)
  balancingSelector3/1 -> [balancing3]
  [balancing4] -> ModuleAssembly4/1(balancing)
  balancingSelector4/1 -> [balancing4]
  [balancing5] -> ModuleAssembly5/1(balancing)
  balancingSelector5/1 -> [balancing5]
  [balancing6] -> ModuleAssembly6/1(balancing)
  balancingSelector6/1 -> [balancing6]
  [balancing7] -> ModuleAssembly7/1(balancing)
  balancingSelector7/1 -> [balancing7]
  [balancing8] -> ModuleAssembly8/1(balancing)
  balancingSelector8/1 -> [balancing8]
  [balancing9] -> ModuleAssembly9/1(balancing)
  balancingSelector9/1 -> [balancing9]
  [balancing10] -> ModuleAssembly10/1(balancing)
  balancingSelector10/1 -> [balancing10]
  CP_ConvBottom_1/1 -> MuxBottom/1
  CP_ConvBottom_2/1 -> MuxBottom/2
  CP_ConvBottom_3/1 -> MuxBottom/3
  MuxBottom/1 -> [CP_OutputsBottom]
  [CP_OutputsBottom] -> CP_Out/1
  connections:
  ModuleAssembly2/LConn1 -- ModuleAssembly1/RConn1
  ModuleAssembly3/LConn1 -- ModuleAssembly2/RConn1
  ModuleAssembly4/LConn1 -- ModuleAssembly3/RConn1
  ModuleAssembly5/LConn1 -- ModuleAssembly4/RConn1
  ModuleAssembly6/LConn1 -- ModuleAssembly5/RConn1
  ModuleAssembly7/LConn1 -- ModuleAssembly6/RConn1
  ModuleAssembly8/LConn1 -- ModuleAssembly7/RConn1
  ModuleAssembly9/LConn1 -- ModuleAssembly8/RConn1
  ModuleAssembly10/LConn1 -- ModuleAssembly9/RConn1
  ModuleAssembly1/LConn1 -- +/RConn1
  ModuleAssembly10/RConn1 -- -/RConn1
  CoolingPlateConnectorBottom/LConn1 -- ModuleAssembly1/RConn2
  CoolingPlateConnectorBottom/LConn2 -- ModuleAssembly2/RConn2
  CoolingPlateConnectorBottom/LConn3 -- ModuleAssembly3/RConn2
  CoolingPlateConnectorBottom/LConn4 -- ModuleAssembly4/RConn2
  CoolingPlateConnectorBottom/LConn5 -- ModuleAssembly5/RConn2
  CoolingPlateConnectorBottom/LConn6 -- ModuleAssembly6/RConn2
  CoolingPlateConnectorBottom/LConn7 -- ModuleAssembly7/RConn2
  CoolingPlateConnectorBottom/LConn8 -- ModuleAssembly8/RConn2
  CoolingPlateConnectorBottom/LConn9 -- ModuleAssembly9/RConn2
  CoolingPlateConnectorBottom/LConn10 -- ModuleAssembly10/RConn2
  CoolingPlateConnectorBottom/RConn1 -- CoolingPlateBottom/LConn2
  FluidIn_To_Bottom/LConn1 -- Fluid_In/RConn1
  Fluid_Out/RConn1 -- FluidOut_From_Bottom/LConn1
  FluidInBottom_From/LConn1 -- CoolingPlateBottom/LConn1
  CoolingPlateBottom/RConn1 -- FluidOutBottom_To/LConn1
  CoolingPlateBottom/RConn2 -- CP_ConvBottom_1/LConn1
  CoolingPlateBottom/RConn3 -- CP_ConvBottom_2/LConn1
  CoolingPlateBottom/RConn4 -- CP_ConvBottom_3/LConn1
